simulink model "ex6"  (R2020b)
settings: Solver=VariableStepAuto  StartTime=0.0  StopTime=10.0  RelTol=1e-3
libraries: fl_lib x69, nesl_utility x2, simulink x1
settings Model: Creator=i7  LastModifiedBy=i7

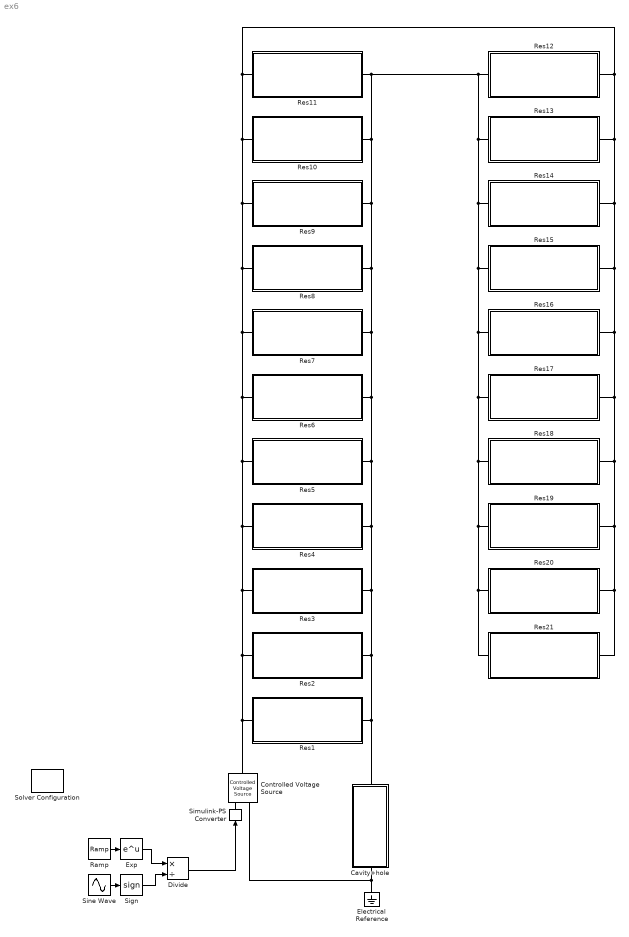
== system ex6 ==
  Cavity+hole : Subsystem
      settings: PortSchema="{\"entries\":[{\"content\":{\"sides\":[{\"content\":{\"connectorIds\":[]},\"type\":\"ConnectorPlacement.EquallySpacedRectSide\",\"uuid\":\"a583a53c-f516-4b69-b36f-f75b7dbb2bb5\"},{\"content\":{\"connectorIds\":[],\"side\":\"RIGHT\"},\"type\":\"ConnectorPlacement.EquallySpacedRectSide\",\"uuid\":\"39101641-aac5-4964-940e-34b93e993ff6\"},{\"content\":{\"connectorIds\":[\"LConn1\"],\"side\":\"TOP\"},\"type\":\"ConnectorPlacement.EquallySpacedRectSide\",\"uuid\":\"c869afa2-0717-4e5a-9ee5-91a1a389dffa\"},{\"content\":{\"connectorIds\":[\"RConn1\"],\"side\":\"BOTTOM\"},\"type\":\"ConnectorPlacement.EquallySpacedRectSide\",\"uuid\":\"edaf248d-6216-4c59-ba6b-fd2e7d02128c\"},{\"content\":{\"connectorIds\":[],\"side\":\"HIDDEN\"},\"type\":\"ConnectorPlacement.EquallySpacedRectSide\",\"uuid\":\"02aea04c-4da5-4e60-9b1a-db560dd0cdf5\"}]},\"type\":\"ConnectorPlacement.EquallySpacedConnector\",\"uuid\":\"1fde798c-4218-4508-966c-7dba91339130\"}],\"packageUris\":[\"http://schema.mathworks.com/mf0/Connector/R2020b\"],\"version\":\"1.0\"}"
  Controlled Voltage Source : fl_lib/Electrical/Electrical Sources/Controlled Voltage Source
  Divide : Product  Inputs=*/
  Electrical Reference : fl_lib/Electrical/Electrical Elements/Electrical Reference
  Exp : Math  SaturateOnIntegerOverflow=on
  Ramp : simulink/Sources/Ramp  slope=-3  start=0  InitialOutput=0
  Res1 : Subsystem
  Res10 : Subsystem
  Res11 : Subsystem
  Res12 : Subsystem
  Res13 : Subsystem
  Res14 : Subsystem
  Res15 : Subsystem
  Res16 : Subsystem
  Res17 : Subsystem
  Res18 : Subsystem
  Res19 : Subsystem
  Res2 : Subsystem
  Res20 : Subsystem
  Res21 : Subsystem
  Res3 : Subsystem
  Res4 : Subsystem
  Res5 : Subsystem
  Res6 : Subsystem
  Res7 : Subsystem
  Res8 : Subsystem
  Res9 : Subsystem
  Sign : Signum
  Simulink-PS Converter : nesl_utility/Simulink-PS Converter  PhysicalDomain=network_engine_domain  SubClassName=ps_input  LeftPortType=input  RightPortType=output  PseudoPeriodic=off  Frequencies=[]  NoiseDistribution=none  NoiseParameters=[]  Unit=1  AffineConversion=off  FilteringAndDerivatives=provide  SimscapeFilterOrder=1  InputFilterTimeConstant=0.001  UdotUserProvided=0
  Sine Wave : Sin  Frequency=2*pi*300  SampleTime=0
  Solver Configuration : nesl_utility/Solver Configuration  PhysicalDomain=network_engine_domain  SubClassName=solver  LeftPortType=input  RightPortType=generic  Tones=[]  Harmonics=[]  SimulateNoise=off  Profile=off  UseLocalSampling=off  EnableSwitchedLinearOptims=on  FrequencyDomain=off  UseCCode=off  RelTol=0.001  AbsTol=1e-06  MinStep=1e-09  ToWorkspace=off  RevertToSquareIcSolve=off  NumHomotopyIterations=100  PhasorMode=off  PhasorModeNumHarmonics=1  DoDC=off  ResidualTolerance=1e-09  UseLocalSolver=off  LocalSolverChoice=NE_BACKWARD_EULER_ADVANCER  LocalSolverSampleTime=0.001  DoFixedCost=off  MaxNonlinIter=3  MaxModeIter=2  ComputeImpulses=off  ImpulseIterations=2  LinearAlgebra=auto  EquationFormulation=NE_TIME_EF  DelaysMemoryBudget=1024  AutomaticFiltering=on  FilteringTimeConstant=0.001  PartitionStorageMethod=AS_NEEDED  PartitionMemoryBudget=1024  PartitionMethod=ROBUST
  wires:
  Ramp/1 -> Exp/1
  Exp/1 -> Divide/1
  Sine Wave/1 -> Sign/1
  Sign/1 -> Divide/2
  Divide/1 -> Simulink-PS Converter/1
  connections:
  Res2/LConn1 -- Res21/LConn1 -- Res20/LConn1 -- Res19/LConn1 -- Res18/LConn1 -- Res17/LConn1 -- Res16/LConn1 -- Res15/LConn1 -- Res14/LConn1 -- Res13/LConn1 -- Res12/LConn1 -- Res11/LConn1 -- Res10/LConn1 -- Res9/LConn1 -- Res8/LConn1 -- Res7/LConn1 -- Res6/LConn1 -- Res5/LConn1 -- Res4/LConn1 -- Res3/LConn1 -- Controlled Voltage Source/LConn1 -- Res1/LConn1
  Res2/RConn1 -- Res21/RConn1 -- Res20/RConn1 -- Res19/RConn1 -- Res18/RConn1 -- Res17/RConn1 -- Res16/RConn1 -- Res15/RConn1 -- Res14/RConn1 -- Res13/RConn1 -- Res12/RConn1 -- Res11/RConn1 -- Res10/RConn1 -- Res9/RConn1 -- Res8/RConn1 -- Res7/RConn1 -- Res6/RConn1 -- Res5/RConn1 -- Res4/RConn1 -- Res3/RConn1 -- Cavity+hole/LConn1 -- Res1/RConn1
  Electrical Reference/LConn1 -- Controlled Voltage Source/RConn2 -- Cavity+hole/RConn1
  Simulink-PS Converter/RConn1 -- Controlled Voltage Source/RConn1

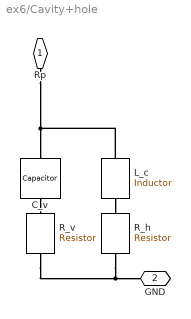
== system ex6/Cavity+hole ==
  C_v : fl_lib/Electrical/Electrical Elements/Capacitor  c=51.919 uF  r=0 Ohm  g=0 1/Ohm  i_specify=off  i_priority=None  i=0 A  i_nominal_specify=off  i_nominal_unit=A  i_nominal_value=1  v_specify=off  v_priority=None  v=0 V  v_nominal_specify=off  v_nominal_unit=V  v_nominal_value=1  vc_specify=off  vc_priority=High  vc=0 V  vc_nominal_specify=off  vc_nominal_unit=V  vc_nominal_value=1
  L_c : fl_lib/Electrical/Electrical Elements/Inductor  l=33.5 mH  r=0 Ohm  g=0 1/Ohm  i_specify=off  i_priority=None  i=0 A  i_nominal_specify=off  i_nominal_unit=A  i_nominal_value=1  v_specify=off  v_priority=None  v=0 V  v_nominal_specify=off  v_nominal_unit=V  v_nominal_value=1  i_L_specify=off  i_L_priority=High  i_L=0 A  i_L_nominal_specify=off  i_L_nominal_unit=A  i_L_nominal_value=1
  R_h : fl_lib/Electrical/Electrical Elements/Resistor  R=0.0969 Ohm  i_specify=off  i_priority=None  i=0 A  i_nominal_specify=off  i_nominal_unit=A  i_nominal_value=1  v_specify=off  v_priority=None  v=0 V  v_nominal_specify=off  v_nominal_unit=V  v_nominal_value=1
  R_v : fl_lib/Electrical/Electrical Elements/Resistor  R=1.4243 Ohm  i_specify=off  i_priority=None  i=0 A  i_nominal_specify=off  i_nominal_unit=A  i_nominal_value=1  v_specify=off  v_priority=None  v=0 V  v_nominal_specify=off  v_nominal_unit=V  v_nominal_value=1
  Rp : PMIOPort  Side=Left
  GND : PMIOPort  Port=2  Side=Right
  connections:
  L_c/LConn1 -- Rp/RConn1 -- C_v/LConn1
  R_h/RConn1 -- R_v/RConn1 -- GND/RConn1
  L_c/RConn1 -- R_h/LConn1
  C_v/RConn1 -- R_v/LConn1

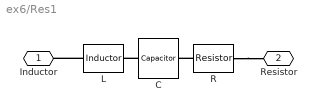
== system ex6/Res1 ==
  C : fl_lib/Electrical/Electrical Elements/Capacitor  c=13.401 uF  r=0 Ohm  g=0 1/Ohm  i_specify=off  i_priority=None  i=0 A  i_nominal_specify=off  i_nominal_unit=A  i_nominal_value=1  v_specify=off  v_priority=None  v=0 V  v_nominal_specify=off  v_nominal_unit=V  v_nominal_value=1  vc_specify=off  vc_priority=High  vc=0 V  vc_nominal_specify=off  vc_nominal_unit=V  vc_nominal_value=1
  L : fl_lib/Electrical/Electrical Elements/Inductor  l=61.3 mH  r=0 Ohm  g=0 1/Ohm  i_specify=off  i_priority=None  i=0 A  i_nominal_specify=off  i_nominal_unit=A  i_nominal_value=1  v_specify=off  v_priority=None  v=0 V  v_nominal_specify=off  v_nominal_unit=V  v_nominal_value=1  i_L_specify=off  i_L_priority=High  i_L=0 A  i_L_nominal_specify=off  i_L_nominal_unit=A  i_L_nominal_value=1
  R : fl_lib/Electrical/Electrical Elements/Resistor  R=1.125 Ohm  i_specify=off  i_priority=None  i=0 A  i_nominal_specify=off  i_nominal_unit=A  i_nominal_value=1  v_specify=off  v_priority=None  v=0 V  v_nominal_specify=off  v_nominal_unit=V  v_nominal_value=1
  Inductor : PMIOPort  Side=Left
  Resistor : PMIOPort  Port=2  Side=Right
  connections:
  R/RConn1 -- Resistor/RConn1
  R/LConn1 -- C/RConn1
  C/LConn1 -- L/RConn1
  L/LConn1 -- Inductor/RConn1

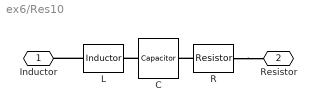
== system ex6/Res10 ==
  C : fl_lib/Electrical/Electrical Elements/Capacitor  c=5.6267 nF  r=0 Ohm  g=0 1/Ohm  i_specify=off  i_priority=None  i=0 A  i_nominal_specify=off  i_nominal_unit=A  i_nominal_value=1  v_specify=off  v_priority=None  v=0 V  v_nominal_specify=off  v_nominal_unit=V  v_nominal_value=1  vc_specify=off  vc_priority=High  vc=0 V  vc_nominal_specify=off  vc_nominal_unit=V  vc_nominal_value=1
  L : fl_lib/Electrical/Electrical Elements/Inductor  l=7500 mH  r=0 Ohm  g=0 1/Ohm  i_specify=off  i_priority=None  i=0 A  i_nominal_specify=off  i_nominal_unit=A  i_nominal_value=1  v_specify=off  v_priority=None  v=0 V  v_nominal_specify=off  v_nominal_unit=V  v_nominal_value=1  i_L_specify=off  i_L_priority=High  i_L=0 A  i_L_nominal_specify=off  i_L_nominal_unit=A  i_L_nominal_value=1
  R : fl_lib/Electrical/Electrical Elements/Resistor  R=400 Ohm  i_specify=off  i_priority=None  i=0 A  i_nominal_specify=off  i_nominal_unit=A  i_nominal_value=1  v_specify=off  v_priority=None  v=0 V  v_nominal_specify=off  v_nominal_unit=V  v_nominal_value=1
  Inductor : PMIOPort  Side=Left
  Resistor : PMIOPort  Port=2  Side=Right
  connections:
  R/RConn1 -- Resistor/RConn1
  R/LConn1 -- C/RConn1
  C/LConn1 -- L/RConn1
  L/LConn1 -- Inductor/RConn1

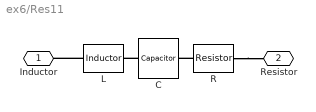
== system ex6/Res11 ==
  C : fl_lib/Electrical/Electrical Elements/Capacitor  c=15.588 nF  r=0 Ohm  g=0 1/Ohm  i_specify=off  i_priority=None  i=0 A  i_nominal_specify=off  i_nominal_unit=A  i_nominal_value=1  v_specify=off  v_priority=None  v=0 V  v_nominal_specify=off  v_nominal_unit=V  v_nominal_value=1  vc_specify=off  vc_priority=High  vc=0 V  vc_nominal_specify=off  vc_nominal_unit=V  vc_nominal_value=1
  L : fl_lib/Electrical/Electrical Elements/Inductor  l=2381 mH  r=0 Ohm  g=0 1/Ohm  i_specify=off  i_priority=None  i=0 A  i_nominal_specify=off  i_nominal_unit=A  i_nominal_value=1  v_specify=off  v_priority=None  v=0 V  v_nominal_specify=off  v_nominal_unit=V  v_nominal_value=1  i_L_specify=off  i_L_priority=High  i_L=0 A  i_L_nominal_specify=off  i_L_nominal_unit=A  i_L_nominal_value=1
  R : fl_lib/Electrical/Electrical Elements/Resistor  R=173.1602 Ohm  i_specify=off  i_priority=None  i=0 A  i_nominal_specify=off  i_nominal_unit=A  i_nominal_value=1  v_specify=off  v_priority=None  v=0 V  v_nominal_specify=off  v_nominal_unit=V  v_nominal_value=1
  Inductor : PMIOPort  Side=Left
  Resistor : PMIOPort  Port=2  Side=Right
  connections:
  R/RConn1 -- Resistor/RConn1
  R/LConn1 -- C/RConn1
  C/LConn1 -- L/RConn1
  L/LConn1 -- Inductor/RConn1

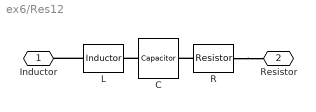
== system ex6/Res12 ==
  C : fl_lib/Electrical/Electrical Elements/Capacitor  c=26.276 nF  r=0 Ohm  g=0 1/Ohm  i_specify=off  i_priority=None  i=0 A  i_nominal_specify=off  i_nominal_unit=A  i_nominal_value=1  v_specify=off  v_priority=None  v=0 V  v_nominal_specify=off  v_nominal_unit=V  v_nominal_value=1  vc_specify=off  vc_priority=High  vc=0 V  vc_nominal_specify=off  vc_nominal_unit=V  vc_nominal_value=1
  L : fl_lib/Electrical/Electrical Elements/Inductor  l=1339.4 mH  r=0 Ohm  g=0 1/Ohm  i_specify=off  i_priority=None  i=0 A  i_nominal_specify=off  i_nominal_unit=A  i_nominal_value=1  v_specify=off  v_priority=None  v=0 V  v_nominal_specify=off  v_nominal_unit=V  v_nominal_value=1  i_L_specify=off  i_L_priority=High  i_L=0 A  i_L_nominal_specify=off  i_L_nominal_unit=A  i_L_nominal_value=1
  R : fl_lib/Electrical/Electrical Elements/Resistor  R=112.3967 Ohm  i_specify=off  i_priority=None  i=0 A  i_nominal_specify=off  i_nominal_unit=A  i_nominal_value=1  v_specify=off  v_priority=None  v=0 V  v_nominal_specify=off  v_nominal_unit=V  v_nominal_value=1
  Inductor : PMIOPort  Side=Left
  Resistor : PMIOPort  Port=2  Side=Right
  connections:
  R/RConn1 -- Resistor/RConn1
  R/LConn1 -- C/RConn1
  C/LConn1 -- L/RConn1
  L/LConn1 -- Inductor/RConn1

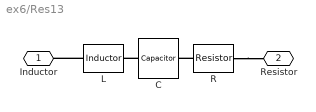
== system ex6/Res13 ==
  C : fl_lib/Electrical/Electrical Elements/Capacitor  c=11.267 nF  r=0 Ohm  g=0 1/Ohm  i_specify=off  i_priority=None  i=0 A  i_nominal_specify=off  i_nominal_unit=A  i_nominal_value=1  v_specify=off  v_priority=None  v=0 V  v_nominal_specify=off  v_nominal_unit=V  v_nominal_value=1  vc_specify=off  vc_priority=High  vc=0 V  vc_nominal_specify=off  vc_nominal_unit=V  vc_nominal_value=1
  L : fl_lib/Electrical/Electrical Elements/Inductor  l=2976.2 mH  r=0 Ohm  g=0 1/Ohm  i_specify=off  i_priority=None  i=0 A  i_nominal_specify=off  i_nominal_unit=A  i_nominal_value=1  v_specify=off  v_priority=None  v=0 V  v_nominal_specify=off  v_nominal_unit=V  v_nominal_value=1  i_L_specify=off  i_L_priority=High  i_L=0 A  i_L_nominal_specify=off  i_L_nominal_unit=A  i_L_nominal_value=1
  R : fl_lib/Electrical/Electrical Elements/Resistor  R=202.0202 Ohm  i_specify=off  i_priority=None  i=0 A  i_nominal_specify=off  i_nominal_unit=A  i_nominal_value=1  v_specify=off  v_priority=None  v=0 V  v_nominal_specify=off  v_nominal_unit=V  v_nominal_value=1
  Inductor : PMIOPort  Side=Left
  Resistor : PMIOPort  Port=2  Side=Right
  connections:
  R/RConn1 -- Resistor/RConn1
  R/LConn1 -- C/RConn1
  C/LConn1 -- L/RConn1
  L/LConn1 -- Inductor/RConn1

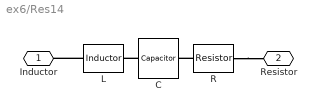
== system ex6/Res14 ==
  C : fl_lib/Electrical/Electrical Elements/Capacitor  c=0.1175 uF  r=0 Ohm  g=0 1/Ohm  i_specify=off  i_priority=None  i=0 A  i_nominal_specify=off  i_nominal_unit=A  i_nominal_value=1  v_specify=off  v_priority=None  v=0 V  v_nominal_specify=off  v_nominal_unit=V  v_nominal_value=1  vc_specify=off  vc_priority=High  vc=0 V  vc_nominal_specify=off  vc_nominal_unit=V  vc_nominal_value=1
  L : fl_lib/Electrical/Electrical Elements/Inductor  l=200 mH  r=0 Ohm  g=0 1/Ohm  i_specify=off  i_priority=None  i=0 A  i_nominal_specify=off  i_nominal_unit=A  i_nominal_value=1  v_specify=off  v_priority=None  v=0 V  v_nominal_specify=off  v_nominal_unit=V  v_nominal_value=1  i_L_specify=off  i_L_priority=High  i_L=0 A  i_L_nominal_specify=off  i_L_nominal_unit=A  i_L_nominal_value=1
  R : fl_lib/Electrical/Electrical Elements/Resistor  R=15 Ohm  i_specify=off  i_priority=None  i=0 A  i_nominal_specify=off  i_nominal_unit=A  i_nominal_value=1  v_specify=off  v_priority=None  v=0 V  v_nominal_specify=off  v_nominal_unit=V  v_nominal_value=1
  Inductor : PMIOPort  Side=Left
  Resistor : PMIOPort  Port=2  Side=Right
  connections:
  R/RConn1 -- Resistor/RConn1
  R/LConn1 -- C/RConn1
  C/LConn1 -- L/RConn1
  L/LConn1 -- Inductor/RConn1

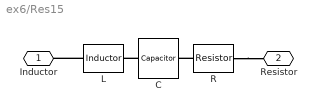
== system ex6/Res15 ==
  C : fl_lib/Electrical/Electrical Elements/Capacitor  c=40.485 nF  r=0 Ohm  g=0 1/Ohm  i_specify=off  i_priority=None  i=0 A  i_nominal_specify=off  i_nominal_unit=A  i_nominal_value=1  v_specify=off  v_priority=None  v=0 V  v_nominal_specify=off  v_nominal_unit=V  v_nominal_value=1  vc_specify=off  vc_priority=High  vc=0 V  vc_nominal_specify=off  vc_nominal_unit=V  vc_nominal_value=1
  L : fl_lib/Electrical/Electrical Elements/Inductor  l=368.7 mH  r=0 Ohm  g=0 1/Ohm  i_specify=off  i_priority=None  i=0 A  i_nominal_specify=off  i_nominal_unit=A  i_nominal_value=1  v_specify=off  v_priority=None  v=0 V  v_nominal_specify=off  v_nominal_unit=V  v_nominal_value=1  i_L_specify=off  i_L_priority=High  i_L=0 A  i_L_nominal_specify=off  i_L_nominal_unit=A  i_L_nominal_value=1
  R : fl_lib/Electrical/Electrical Elements/Resistor  R=58.651 Ohm  i_specify=off  i_priority=None  i=0 A  i_nominal_specify=off  i_nominal_unit=A  i_nominal_value=1  v_specify=off  v_priority=None  v=0 V  v_nominal_specify=off  v_nominal_unit=V  v_nominal_value=1
  Inductor : PMIOPort  Side=Left
  Resistor : PMIOPort  Port=2  Side=Right
  connections:
  R/RConn1 -- Resistor/RConn1
  R/LConn1 -- C/RConn1
  C/LConn1 -- L/RConn1
  L/LConn1 -- Inductor/RConn1

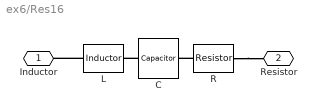
== system ex6/Res16 ==
  C : fl_lib/Electrical/Electrical Elements/Capacitor  c=28.792 F  r=0 Ohm  g=0 1/Ohm  i_specify=off  i_priority=None  i=0 A  i_nominal_specify=off  i_nominal_unit=A  i_nominal_value=1  v_specify=off  v_priority=None  v=0 V  v_nominal_specify=off  v_nominal_unit=V  v_nominal_value=1  vc_specify=off  vc_priority=High  vc=0 V  vc_nominal_specify=off  vc_nominal_unit=V  vc_nominal_value=1
  L : fl_lib/Electrical/Electrical Elements/Inductor  l=491.2 mH  r=0 Ohm  g=0 1/Ohm  i_specify=off  i_priority=None  i=0 A  i_nominal_specify=off  i_nominal_unit=A  i_nominal_value=1  v_specify=off  v_priority=None  v=0 V  v_nominal_specify=off  v_nominal_unit=V  v_nominal_value=1  i_L_specify=off  i_L_priority=High  i_L=0 A  i_L_nominal_specify=off  i_L_nominal_unit=A  i_L_nominal_value=1
  R : fl_lib/Electrical/Electrical Elements/Resistor  R=491.2 Ohm  i_specify=off  i_priority=None  i=0 A  i_nominal_specify=off  i_nominal_unit=A  i_nominal_value=1  v_specify=off  v_priority=None  v=0 V  v_nominal_specify=off  v_nominal_unit=V  v_nominal_value=1
  Inductor : PMIOPort  Side=Left
  Resistor : PMIOPort  Port=2  Side=Right
  connections:
  R/RConn1 -- Resistor/RConn1
  R/LConn1 -- C/RConn1
  C/LConn1 -- L/RConn1
  L/LConn1 -- Inductor/RConn1

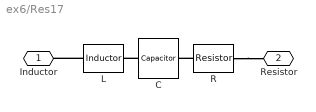
== system ex6/Res17 ==
  C : fl_lib/Electrical/Electrical Elements/Capacitor  c=59.5 nF  r=0 Ohm  g=0 1/Ohm  i_specify=off  i_priority=None  i=0 A  i_nominal_specify=off  i_nominal_unit=A  i_nominal_value=1  v_specify=off  v_priority=None  v=0 V  v_nominal_specify=off  v_nominal_unit=V  v_nominal_value=1  vc_specify=off  vc_priority=High  vc=0 V  vc_nominal_specify=off  vc_nominal_unit=V  vc_nominal_value=1
  L : fl_lib/Electrical/Electrical Elements/Inductor  l=200 mH  r=0 Ohm  g=0 1/Ohm  i_specify=off  i_priority=None  i=0 A  i_nominal_specify=off  i_nominal_unit=A  i_nominal_value=1  v_specify=off  v_priority=None  v=0 V  v_nominal_specify=off  v_nominal_unit=V  v_nominal_value=1  i_L_specify=off  i_L_priority=High  i_L=0 A  i_L_nominal_specify=off  i_L_nominal_unit=A  i_L_nominal_value=1
  R : fl_lib/Electrical/Electrical Elements/Resistor  R=27 Ohm  i_specify=off  i_priority=None  i=0 A  i_nominal_specify=off  i_nominal_unit=A  i_nominal_value=1  v_specify=off  v_priority=None  v=0 V  v_nominal_specify=off  v_nominal_unit=V  v_nominal_value=1
  Inductor : PMIOPort  Side=Left
  Resistor : PMIOPort  Port=2  Side=Right
  connections:
  R/RConn1 -- Resistor/RConn1
  R/LConn1 -- C/RConn1
  C/LConn1 -- L/RConn1
  L/LConn1 -- Inductor/RConn1

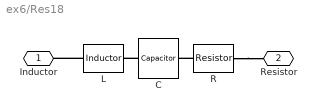
== system ex6/Res18 ==
  C : fl_lib/Electrical/Electrical Elements/Capacitor  c=20.865 nF  r=0 Ohm  g=0 1/Ohm  i_specify=off  i_priority=None  i=0 A  i_nominal_specify=off  i_nominal_unit=A  i_nominal_value=1  v_specify=off  v_priority=None  v=0 V  v_nominal_specify=off  v_nominal_unit=V  v_nominal_value=1  vc_specify=off  vc_priority=High  vc=0 V  vc_nominal_specify=off  vc_nominal_unit=V  vc_nominal_value=1
  L : fl_lib/Electrical/Electrical Elements/Inductor  l=520.8 mH  r=0 Ohm  g=0 1/Ohm  i_specify=off  i_priority=None  i=0 A  i_nominal_specify=off  i_nominal_unit=A  i_nominal_value=1  v_specify=off  v_priority=None  v=0 V  v_nominal_specify=off  v_nominal_unit=V  v_nominal_value=1  i_L_specify=off  i_L_priority=High  i_L=0 A  i_L_nominal_specify=off  i_L_nominal_unit=A  i_L_nominal_value=1
  R : fl_lib/Electrical/Electrical Elements/Resistor  R=61.3636 Ohm  i_specify=off  i_priority=None  i=0 A  i_nominal_specify=off  i_nominal_unit=A  i_nominal_value=1  v_specify=off  v_priority=None  v=0 V  v_nominal_specify=off  v_nominal_unit=V  v_nominal_value=1
  Inductor : PMIOPort  Side=Left
  Resistor : PMIOPort  Port=2  Side=Right
  connections:
  R/RConn1 -- Resistor/RConn1
  R/LConn1 -- C/RConn1
  C/LConn1 -- L/RConn1
  L/LConn1 -- Inductor/RConn1

== system ex6/Res19 ==
  C : fl_lib/Electrical/Electrical Elements/Capacitor  c=3.978 nF  r=0 Ohm  g=0 1/Ohm  i_specify=off  i_priority=None  i=0 A  i_nominal_specify=off  i_nominal_unit=A  i_nominal_value=1  v_specify=off  v_priority=None  v=0 V  v_nominal_specify=off  v_nominal_unit=V  v_nominal_value=1  vc_specify=off  vc_priority=High  vc=0 V  vc_nominal_specify=off  vc_nominal_unit=V  vc_nominal_value=1
  L : fl_lib/Electrical/Electrical Elements/Inductor  l=2564.1 mH  r=0 Ohm  g=0 1/Ohm  i_specify=off  i_priority=None  i=0 A  i_nominal_specify=off  i_nominal_unit=A  i_nominal_value=1  v_specify=off  v_priority=None  v=0 V  v_nominal_specify=off  v_nominal_unit=V  v_nominal_value=1  i_L_specify=off  i_L_priority=High  i_L=0 A  i_L_nominal_specify=off  i_L_nominal_unit=A  i_L_nominal_value=1
  R : fl_lib/Electrical/Electrical Elements/Resistor  R=377.6777 Ohm  i_specify=off  i_priority=None  i=0 A  i_nominal_specify=off  i_nominal_unit=A  i_nominal_value=1  v_specify=off  v_priority=None  v=0 V  v_nominal_specify=off  v_nominal_unit=V  v_nominal_value=1
  Inductor : PMIOPort  Side=Left
  Resistor : PMIOPort  Port=2  Side=Right
  connections:
  R/RConn1 -- Resistor/RConn1
  R/LConn1 -- C/RConn1
  C/LConn1 -- L/RConn1
  L/LConn1 -- Inductor/RConn1

== system ex6/Res2 ==
  C : fl_lib/Electrical/Electrical Elements/Capacitor  c=0.58997 uF  r=0 Ohm  g=0 1/Ohm  i_specify=off  i_priority=None  i=0 A  i_nominal_specify=off  i_nominal_unit=A  i_nominal_value=1  v_specify=off  v_priority=None  v=0 V  v_nominal_specify=off  v_nominal_unit=V  v_nominal_value=1  vc_specify=off  vc_priority=High  vc=0 V  vc_nominal_specify=off  vc_nominal_unit=V  vc_nominal_value=1
  L : fl_lib/Electrical/Electrical Elements/Inductor  l=779.6 mH  r=0 Ohm  g=0 1/Ohm  i_specify=off  i_priority=None  i=0 A  i_nominal_specify=off  i_nominal_unit=A  i_nominal_value=1  v_specify=off  v_priority=None  v=0 V  v_nominal_specify=off  v_nominal_unit=V  v_nominal_value=1  i_L_specify=off  i_L_priority=High  i_L=0 A  i_L_nominal_specify=off  i_L_nominal_unit=A  i_L_nominal_value=1
  R : fl_lib/Electrical/Electrical Elements/Resistor  R=1 Ohm  i_specify=off  i_priority=None  i=0 A  i_nominal_specify=off  i_nominal_unit=A  i_nominal_value=1  v_specify=off  v_priority=None  v=0 V  v_nominal_specify=off  v_nominal_unit=V  v_nominal_value=1
  Resistor : PMIOPort  Port=2  Side=Right
  Inductor : PMIOPort  Side=Left
  connections:
  R/RConn1 -- Resistor/RConn1
  R/LConn1 -- C/RConn1
  C/LConn1 -- L/RConn1
  L/LConn1 -- Inductor/RConn1

== system ex6/Res20 ==
  C : fl_lib/Electrical/Electrical Elements/Capacitor  c=7.533 nF  r=0 Ohm  g=0 1/Ohm  i_specify=off  i_priority=None  i=0 A  i_nominal_specify=off  i_nominal_unit=A  i_nominal_value=1  v_specify=off  v_priority=None  v=0 V  v_nominal_specify=off  v_nominal_unit=V  v_nominal_value=1  vc_specify=off  vc_priority=High  vc=0 V  vc_nominal_specify=off  vc_nominal_unit=V  vc_nominal_value=1
  L : fl_lib/Electrical/Electrical Elements/Inductor  l=1039 mH  r=0 Ohm  g=0 1/Ohm  i_specify=off  i_priority=None  i=0 A  i_nominal_specify=off  i_nominal_unit=A  i_nominal_value=1  v_specify=off  v_priority=None  v=0 V  v_nominal_specify=off  v_nominal_unit=V  v_nominal_value=1  i_L_specify=off  i_L_priority=High  i_L=0 A  i_L_nominal_specify=off  i_L_nominal_unit=A  i_L_nominal_value=1
  R : fl_lib/Electrical/Electrical Elements/Resistor  R=158.6777 Ohm  i_specify=off  i_priority=None  i=0 A  i_nominal_specify=off  i_nominal_unit=A  i_nominal_value=1  v_specify=off  v_priority=None  v=0 V  v_nominal_specify=off  v_nominal_unit=V  v_nominal_value=1
  Inductor : PMIOPort  Side=Left
  Resistor : PMIOPort  Port=2  Side=Right
  connections:
  R/RConn1 -- Resistor/RConn1
  R/LConn1 -- C/RConn1
  C/LConn1 -- L/RConn1
  L/LConn1 -- Inductor/RConn1

== system ex6/Res21 ==
  C : fl_lib/Electrical/Electrical Elements/Capacitor  c=10.067 nF  r=0 Ohm  g=0 1/Ohm  i_specify=off  i_priority=None  i=0 A  i_nominal_specify=off  i_nominal_unit=A  i_nominal_value=1  v_specify=off  v_priority=None  v=0 V  v_nominal_specify=off  v_nominal_unit=V  v_nominal_value=1  vc_specify=off  vc_priority=High  vc=0 V  vc_nominal_specify=off  vc_nominal_unit=V  vc_nominal_value=1
  L : fl_lib/Electrical/Electrical Elements/Inductor  l=750 mH  r=0 Ohm  g=0 1/Ohm  i_specify=off  i_priority=None  i=0 A  i_nominal_specify=off  i_nominal_unit=A  i_nominal_value=1  v_specify=off  v_priority=None  v=0 V  v_nominal_specify=off  v_nominal_unit=V  v_nominal_value=1  i_L_specify=off  i_L_priority=High  i_L=0 A  i_L_nominal_specify=off  i_L_nominal_unit=A  i_L_nominal_value=1
  R : fl_lib/Electrical/Electrical Elements/Resistor  R=122.7273 Ohm  i_specify=off  i_priority=None  i=0 A  i_nominal_specify=off  i_nominal_unit=A  i_nominal_value=1  v_specify=off  v_priority=None  v=0 V  v_nominal_specify=off  v_nominal_unit=V  v_nominal_value=1
  Inductor : PMIOPort  Side=Left
  Resistor : PMIOPort  Port=2  Side=Right
  connections:
  R/RConn1 -- Resistor/RConn1
  R/LConn1 -- C/RConn1
  C/LConn1 -- L/RConn1
  L/LConn1 -- Inductor/RConn1

== system ex6/Res3 ==
  C : fl_lib/Electrical/Electrical Elements/Capacitor  c=0.39276 uF  r=0 Ohm  g=0 1/Ohm  i_specify=off  i_priority=None  i=0 A  i_nominal_specify=off  i_nominal_unit=A  i_nominal_value=1  v_specify=off  v_priority=None  v=0 V  v_nominal_specify=off  v_nominal_unit=V  v_nominal_value=1  vc_specify=off  vc_priority=High  vc=0 V  vc_nominal_specify=off  vc_nominal_unit=V  vc_nominal_value=1
  L : fl_lib/Electrical/Electrical Elements/Inductor  l=333.5 mH  r=0 Ohm  g=0 1/Ohm  i_specify=off  i_priority=None  i=0 A  i_nominal_specify=off  i_nominal_unit=A  i_nominal_value=1  v_specify=off  v_priority=None  v=0 V  v_nominal_specify=off  v_nominal_unit=V  v_nominal_value=1  i_L_specify=off  i_L_priority=High  i_L=0 A  i_L_nominal_specify=off  i_L_nominal_unit=A  i_L_nominal_value=1
  R : fl_lib/Electrical/Electrical Elements/Resistor  R=20.8579 Ohm  i_specify=off  i_priority=None  i=0 A  i_nominal_specify=off  i_nominal_unit=A  i_nominal_value=1  v_specify=off  v_priority=None  v=0 V  v_nominal_specify=off  v_nominal_unit=V  v_nominal_value=1
  Inductor : PMIOPort  Side=Left
  Resistor : PMIOPort  Port=2  Side=Right
  connections:
  R/RConn1 -- Resistor/RConn1
  R/LConn1 -- C/RConn1
  C/LConn1 -- L/RConn1
  L/LConn1 -- Inductor/RConn1

== system ex6/Res4 ==
  C : fl_lib/Electrical/Electrical Elements/Capacitor  c=0.16493 uF  r=0 Ohm  g=0 1/Ohm  i_specify=off  i_priority=None  i=0 A  i_nominal_specify=off  i_nominal_unit=A  i_nominal_value=1  v_specify=off  v_priority=None  v=0 V  v_nominal_specify=off  v_nominal_unit=V  v_nominal_value=1  vc_specify=off  vc_priority=High  vc=0 V  vc_nominal_specify=off  vc_nominal_unit=V  vc_nominal_value=1
  L : fl_lib/Electrical/Electrical Elements/Inductor  l=607.6 mH  r=0 Ohm  g=0 1/Ohm  i_specify=off  i_priority=None  i=0 A  i_nominal_specify=off  i_nominal_unit=A  i_nominal_value=1  v_specify=off  v_priority=None  v=0 V  v_nominal_specify=off  v_nominal_unit=V  v_nominal_value=1  i_L_specify=off  i_L_priority=High  i_L=0 A  i_L_nominal_specify=off  i_L_nominal_unit=A  i_L_nominal_value=1
  R : fl_lib/Electrical/Electrical Elements/Resistor  R=31.8235 Ohm  i_specify=off  i_priority=None  i=0 A  i_nominal_specify=off  i_nominal_unit=A  i_nominal_value=1  v_specify=off  v_priority=None  v=0 V  v_nominal_specify=off  v_nominal_unit=V  v_nominal_value=1
  Inductor : PMIOPort  Side=Left
  Resistor : PMIOPort  Port=2  Side=Right
  connections:
  R/RConn1 -- Resistor/RConn1
  R/LConn1 -- C/RConn1
  C/LConn1 -- L/RConn1
  L/LConn1 -- Inductor/RConn1

== system ex6/Res5 ==
  C : fl_lib/Electrical/Electrical Elements/Capacitor  c=44.557 nF  r=0 Ohm  g=0 1/Ohm  i_specify=off  i_priority=None  i=0 A  i_nominal_specify=off  i_nominal_unit=A  i_nominal_value=1  v_specify=off  v_priority=None  v=0 V  v_nominal_specify=off  v_nominal_unit=V  v_nominal_value=1  vc_specify=off  vc_priority=High  vc=0 V  vc_nominal_specify=off  vc_nominal_unit=V  vc_nominal_value=1
  L : fl_lib/Electrical/Electrical Elements/Inductor  l=1961.5 mH  r=0 Ohm  g=0 1/Ohm  i_specify=off  i_priority=None  i=0 A  i_nominal_specify=off  i_nominal_unit=A  i_nominal_value=1  v_specify=off  v_priority=None  v=0 V  v_nominal_specify=off  v_nominal_unit=V  v_nominal_value=1  i_L_specify=off  i_L_priority=High  i_L=0 A  i_L_nominal_specify=off  i_L_nominal_unit=A  i_L_nominal_value=1
  R : fl_lib/Electrical/Electrical Elements/Resistor  R=63.4615 Ohm  i_specify=off  i_priority=None  i=0 A  i_nominal_specify=off  i_nominal_unit=A  i_nominal_value=1  v_specify=off  v_priority=None  v=0 V  v_nominal_specify=off  v_nominal_unit=V  v_nominal_value=1
  Inductor : PMIOPort  Side=Left
  Resistor : PMIOPort  Port=2  Side=Right
  connections:
  R/RConn1 -- Resistor/RConn1
  R/LConn1 -- C/RConn1
  C/LConn1 -- L/RConn1
  L/LConn1 -- Inductor/RConn1

== system ex6/Res6 ==
  C : fl_lib/Electrical/Electrical Elements/Capacitor  c=47.828 F  r=0 Ohm  g=0 1/Ohm  i_specify=off  i_priority=None  i=0 A  i_nominal_specify=off  i_nominal_unit=A  i_nominal_value=1  v_specify=off  v_priority=None  v=0 V  v_nominal_specify=off  v_nominal_unit=V  v_nominal_value=1  vc_specify=off  vc_priority=High  vc=0 V  vc_nominal_specify=off  vc_nominal_unit=V  vc_nominal_value=1
  L : fl_lib/Electrical/Electrical Elements/Inductor  l=1500 mH  r=0 Ohm  g=0 1/Ohm  i_specify=off  i_priority=None  i=0 A  i_nominal_specify=off  i_nominal_unit=A  i_nominal_value=1  v_specify=off  v_priority=None  v=0 V  v_nominal_specify=off  v_nominal_unit=V  v_nominal_value=1  i_L_specify=off  i_L_priority=High  i_L=0 A  i_L_nominal_specify=off  i_L_nominal_unit=A  i_L_nominal_value=1
  R : fl_lib/Electrical/Electrical Elements/Resistor  R=80.8824 Ohm  i_specify=off  i_priority=None  i=0 A  i_nominal_specify=off  i_nominal_unit=A  i_nominal_value=1  v_specify=off  v_priority=None  v=0 V  v_nominal_specify=off  v_nominal_unit=V  v_nominal_value=1
  Inductor : PMIOPort  Side=Left
  Resistor : PMIOPort  Port=2  Side=Right
  connections:
  R/RConn1 -- Resistor/RConn1
  R/LConn1 -- C/RConn1
  C/LConn1 -- L/RConn1
  L/LConn1 -- Inductor/RConn1

== system ex6/Res7 ==
  C : fl_lib/Electrical/Electrical Elements/Capacitor  c=48.677 nF  r=0 Ohm  g=0 1/Ohm  i_specify=off  i_priority=None  i=0 A  i_nominal_specify=off  i_nominal_unit=A  i_nominal_value=1  v_specify=off  v_priority=None  v=0 V  v_nominal_specify=off  v_nominal_unit=V  v_nominal_value=1  vc_specify=off  vc_priority=High  vc=0 V  vc_nominal_specify=off  vc_nominal_unit=V  vc_nominal_value=1
  L : fl_lib/Electrical/Electrical Elements/Inductor  l=1375 mH  r=0 Ohm  g=0 1/Ohm  i_specify=off  i_priority=None  i=0 A  i_nominal_specify=off  i_nominal_unit=A  i_nominal_value=1  v_specify=off  v_priority=None  v=0 V  v_nominal_specify=off  v_nominal_unit=V  v_nominal_value=1  i_L_specify=off  i_L_priority=High  i_L=0 A  i_L_nominal_specify=off  i_L_nominal_unit=A  i_L_nominal_value=1
  R : fl_lib/Electrical/Electrical Elements/Resistor  R=110 Ohm  i_specify=off  i_priority=None  i=0 A  i_nominal_specify=off  i_nominal_unit=A  i_nominal_value=1  v_specify=off  v_priority=None  v=0 V  v_nominal_specify=off  v_nominal_unit=V  v_nominal_value=1
  Inductor : PMIOPort  Side=Left
  Resistor : PMIOPort  Port=2  Side=Right
  connections:
  R/RConn1 -- Resistor/RConn1
  R/LConn1 -- C/RConn1
  C/LConn1 -- L/RConn1
  L/LConn1 -- Inductor/RConn1

== system ex6/Res8 ==
  C : fl_lib/Electrical/Electrical Elements/Capacitor  c=0.1216 uF  r=0 Ohm  g=0 1/Ohm  i_specify=off  i_priority=None  i=0 A  i_nominal_specify=off  i_nominal_unit=A  i_nominal_value=1  v_specify=off  v_priority=None  v=0 V  v_nominal_specify=off  v_nominal_unit=V  v_nominal_value=1  vc_specify=off  vc_priority=High  vc=0 V  vc_nominal_specify=off  vc_nominal_unit=V  vc_nominal_value=1
  L : fl_lib/Electrical/Electrical Elements/Inductor  l=500 mH  r=0 Ohm  g=0 1/Ohm  i_specify=off  i_priority=None  i=0 A  i_nominal_specify=off  i_nominal_unit=A  i_nominal_value=1  v_specify=off  v_priority=None  v=0 V  v_nominal_specify=off  v_nominal_unit=V  v_nominal_value=1  i_L_specify=off  i_L_priority=High  i_L=0 A  i_L_nominal_specify=off  i_L_nominal_unit=A  i_L_nominal_value=1
  R : fl_lib/Electrical/Electrical Elements/Resistor  R=31 Ohm  i_specify=off  i_priority=None  i=0 A  i_nominal_specify=off  i_nominal_unit=A  i_nominal_value=1  v_specify=off  v_priority=None  v=0 V  v_nominal_specify=off  v_nominal_unit=V  v_nominal_value=1
  Inductor : PMIOPort  Side=Left
  Resistor : PMIOPort  Port=2  Side=Right
  connections:
  R/RConn1 -- Resistor/RConn1
  R/LConn1 -- C/RConn1
  C/LConn1 -- L/RConn1
  L/LConn1 -- Inductor/RConn1

== system ex6/Res9 ==
  C : fl_lib/Electrical/Electrical Elements/Capacitor  c=6.4 nF  r=0 Ohm  g=0 1/Ohm  i_specify=off  i_priority=None  i=0 A  i_nominal_specify=off  i_nominal_unit=A  i_nominal_value=1  v_specify=off  v_priority=None  v=0 V  v_nominal_specify=off  v_nominal_unit=V  v_nominal_value=1  vc_specify=off  vc_priority=High  vc=0 V  vc_nominal_specify=off  vc_nominal_unit=V  vc_nominal_value=1
  L : fl_lib/Electrical/Electrical Elements/Inductor  l=7500 mH  r=0 Ohm  g=0 1/Ohm  i_specify=off  i_priority=None  i=0 A  i_nominal_specify=off  i_nominal_unit=A  i_nominal_value=1  v_specify=off  v_priority=None  v=0 V  v_nominal_specify=off  v_nominal_unit=V  v_nominal_value=1  i_L_specify=off  i_L_priority=High  i_L=0 A  i_L_nominal_specify=off  i_L_nominal_unit=A  i_L_nominal_value=1
  R : fl_lib/Electrical/Electrical Elements/Resistor  R=400 Ohm  i_specify=off  i_priority=None  i=0 A  i_nominal_specify=off  i_nominal_unit=A  i_nominal_value=1  v_specify=off  v_priority=None  v=0 V  v_nominal_specify=off  v_nominal_unit=V  v_nominal_value=1
  Inductor : PMIOPort  Side=Left
  Resistor : PMIOPort  Port=2  Side=Right
  connections:
  R/RConn1 -- Resistor/RConn1
  R/LConn1 -- C/RConn1
  C/LConn1 -- L/RConn1
  L/LConn1 -- Inductor/RConn1
